simulink model "Project5Simulink"  (R2020a)
settings: Solver=VariableStepAuto  StartTime=0.0  StopTime=10.0  MaxStep=0.01  RelTol=1e-3
values from neighbouring files (symbols this model uses):
  b = 0.3    [Project4.m]    (also in Project5.m = 1)
  F = 1    [Project4.m]    (also in Project5.m = 10)
  k = 20    [Project4.m]    (also in Project5.m)
  M = 1    [Project4.m]    (also in Project5.m)
settings Model: Creator=cresp  LastModifiedBy=cresp

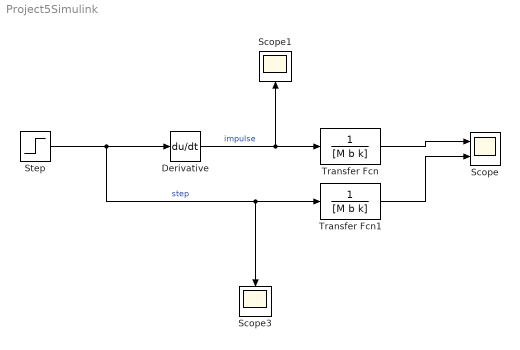
== system Project5Simulink ==
  Derivative : Derivative
  Scope : Scope  NumInputPorts=2
  Scope1 : Scope
  Scope3 : Scope
  Step : Step  After=F  SampleTime=0
  Transfer Fcn : TransferFcn  Denominator=[M b k]
  Transfer Fcn1 : TransferFcn  Denominator=[M b k]
  wires:
  Transfer Fcn/1 -> Scope/1
  Step/1 -> Scope3/1, Transfer Fcn1/1, Derivative/1  "step"
  Derivative/1 -> Transfer Fcn/1, Scope1/1  "impulse"
  Transfer Fcn1/1 -> Scope/2
